simulink model "a1"  (Simulink 8.7)
settings: Solver=ode45  StartTime=0.0  StopTime=5555  RelTol=1e-3
settings Model: Creator=birger  LastModifiedBy=Birger
settings DataIOCC: LimitDataPoints=off  SaveFormat=Dataset
settings DebuggingCC: UnderspecifiedInitializationDetection=Simplified  MergeDetectMultiDrivingBlocksExec=error
settings HardwareCC: ProdBitPerPointer=64  ProdLargestAtomicFloat=Float  ProdIntDivRoundTo=Zero  ProdEndianess=LittleEndian  ProdWordSize=64  ProdHWDeviceType=Intel->x86-64 (Windows64)
settings ModelReferenceCC: PropagateSignalLabelsOutOfModel=on
settings ConfigComp: CovModelRefEnable=off

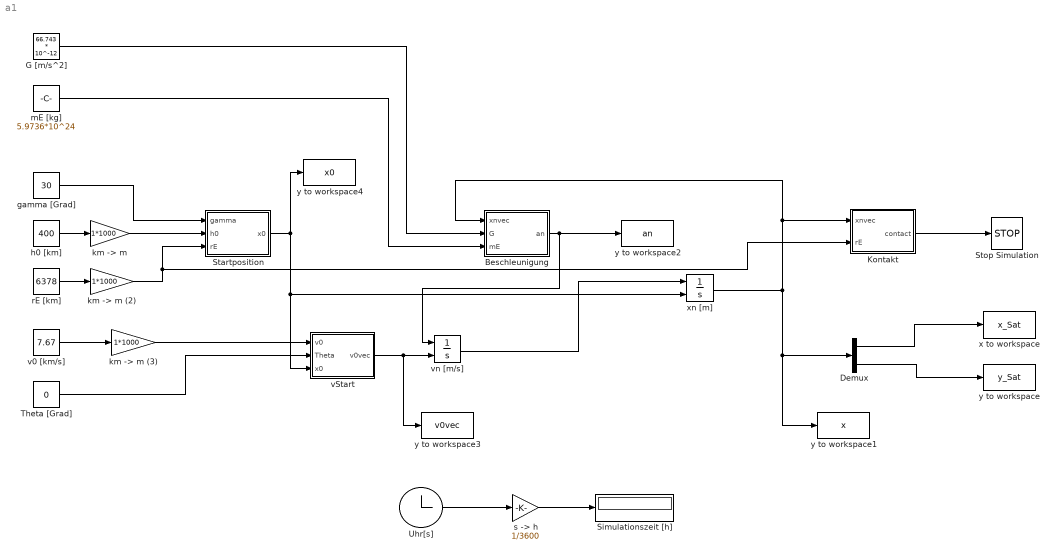
== system a1 ==
  Beschleunigung : MATLAB Function  TreatAsAtomicUnit=on
  Demux : Demux  Outputs=2
  G [m/s^2] : Constant  Value=66.743 * 10^-12
  Kontakt : MATLAB Function  TreatAsAtomicUnit=on
  "Simulationszeit [h] " : Display
  Startposition : MATLAB Function  TreatAsAtomicUnit=on
  Stop Simulation : Stop
  Theta [Grad] : Constant  Value=0
  Uhr[s] : Clock
  gamma [Grad] : Constant  Value=30
  h0 [km] : Constant  Value=400
  "km -> m" : Gain  Gain=1*1000
  "km -> m (2)" : Gain  Gain=1*1000
  "km -> m (3)" : Gain  Gain=1*1000
  mE [kg] : Constant  Value=5.9736*10^24
  rE [km] : Constant  Value=6378
  "s -> h" : Gain  Gain=1/3600
  v0 [km/s] : Constant  Value=7.67
  vStart : MATLAB Function  TreatAsAtomicUnit=on
  vn [m/s] : Integrator  InitialConditionSource=external
  x to workspace : ToWorkspace  VariableName=x_Sat  SampleTime=-1
  xn [m] : Integrator  InitialConditionSource=external
  y to workspace : ToWorkspace  VariableName=y_Sat  SampleTime=-1
  y to workspace1 : ToWorkspace  VariableName=x  SampleTime=-1
  y to workspace2 : ToWorkspace  VariableName=an  SampleTime=-1
  y to workspace3 : ToWorkspace  VariableName=v0vec  SampleTime=-1
  y to workspace4 : ToWorkspace  VariableName=x0  SampleTime=-1
  wires:
  Kontakt/1(contact) -> Stop Simulation/1
  Demux/1 -> x to workspace/1
  Demux/2 -> y to workspace/1
  gamma [Grad]/1 -> Startposition/1(gamma)
  Theta [Grad]/1 -> vStart/2(Theta)
  Startposition/1(x0) -> xn [m]/2, vStart/3(x0), y to workspace4/1
  vStart/1(v0vec) -> y to workspace3/1, vn [m/s]/2
  xn [m]/1 -> Kontakt/1(xnvec), Beschleunigung/1(xnvec), y to workspace1/1, Demux/1
  Beschleunigung/1(an) -> y to workspace2/1, vn [m/s]/1
  mE [kg]/1 -> Beschleunigung/3(mE)
  G [m/s^2]/1 -> Beschleunigung/2(G)
  vn [m/s]/1 -> xn [m]/1
  Uhr[s]/1 -> "s -> h"/1
  "s -> h"/1 -> "Simulationszeit [h] "/1
  h0 [km]/1 -> "km -> m"/1
  "km -> m"/1 -> Startposition/2(h0)
  "km -> m (2)"/1 -> Kontakt/2(rE), Startposition/3(rE)
  rE [km]/1 -> "km -> m (2)"/1
  "km -> m (3)"/1 -> vStart/1(v0)
  v0 [km/s]/1 -> "km -> m (3)"/1

== matlab function vStart ==
  data: v0 input double; v0vec output double; Theta input double; x0 input double
function v0vec = fcn(v0,Theta,x0)

%Einheitsvektoren n und t
n = x0 / norm(x0);  %x0 auf Laenge 1
t = [n(2); -n(1)]; %senkrecht auf x0 mit Laenge 1

%Komponenten vn und vt
vt = v0 * cosd(Theta);
vn = v0 * sind(Theta);

%v0Welt aus laenge * richtung (in m/s)
v0vec = (vt * t) + (vn * n);

== matlab function Startposition ==
  data: gamma input double; x0 output double; h0 input double; rE input double
function x0 = fcn(gamma,h0,rE)

r = rE + h0; %Hypothenuse
x0 = [cosd(gamma) * r ; sind(gamma) * r ];

== matlab function Beschleunigung ==
  data: xnvec input double; an output double; G input double; mE input double
function an = fcn(xnvec,G,mE)
%#codegen

%r und eSE berechnen
r = norm(xnvec);
eSE = -xnvec / r;

%Beschleunigung berechnen
an = G * (mE / r^2) * eSE;

== matlab function Kontakt ==
  data: xnvec input double; contact output double; rE input double
function contact = fcn(xnvec,rE)
%#codegen

rSE = norm(xnvec);
h = rSE - rE;

if h > 0
    contact = 0;
else
    contact = 1;
end
